simulink model "Galvo_sys_cc_neu_v32"  (R2013a)
settings: Solver=ode45  StartTime=0.0  StopTime=5e-3  MaxStep=1e-4  RelTol=1e-3  AbsTol=1e-5
PreLoadFcn:
  | paramCtrl=evalin('base','paramCtrl;');
  | 
  | I_LIM=str2num(paramCtrl.I_LIM);
  | Kbc=str2num(paramCtrl.Kbc);
InitFcn:
  | %I_LIM=str2num(paramCtrl.I_LIM);
  | %Kbc=str2num(paramCtrl.Kbc);
StartFcn:
  | %I_LIM=str2num(paramCtrl.I_LIM);
  | %Kbc=str2num(paramCtrl.Kbc);
values from neighbouring files (symbols this model uses):
  Lc = 170e-6    (= 0.00017)    [Galvo_process_analyze.m]
  Rc = 1.5    [Galvo_process_analyze.m]
undefined symbols (not defined in the file or in its folder): Rsh
libraries: simulink x2
settings Model: BufferReuse=off  Creator=mainster  LastModifiedBy=mainster
settings OptimizationCC: BlockReduction=off  OptimizeBlockIOStorage=off  BufferReuse=off  ExpressionFolding=off  LocalBlockOutputs=off
settings ModelReferenceCC: ModelReferenceNumInstancesAllowed=Single

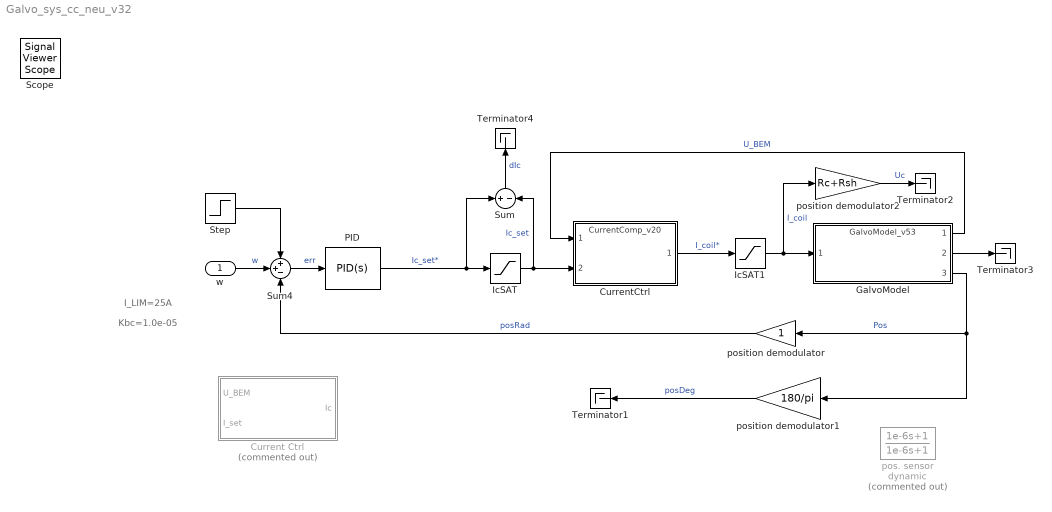
== system Galvo_sys_cc_neu_v32 ==
  note: I_LIM=25A
  note: Kbc=1.0e-05
  w : Inport
  Current Ctrl : Subsystem  Commented=on
  CurrentCtrl : ModelReference  ModelNameDialog=CurrentComp_v20.slx  SimulationMode=Normal  Variant=on  OverrideUsingVariant=cc_v20  ModelReferenceVersion=1.87  CopyOfModelName=CurrentComp_v20.slx  DefaultDataLogging=on
      mask Display:
      | str=sprintf('%s',get(gcbh,'ModelName'));
      | port_label('input', 2, 'I_{Set Coil}','texmode','on')
      | color('red');
      | port_label('input', 1, 'U_{BEM}','texmode','on')
      | color('black');
      | port_label('output', 1, 'I_{Coil}','texmode','on')
      | %text(.05,.98,['{\fontsize{12}\it\bf' strrep(str,'_',' ') '}'],'horizontalAlignment','left','verticalAlignment','top','texmode','on')
      | text(.95,0.95,['{\fontsize{12}\it\bfG_{cc}(s)}'],'horizontalAlignment','right','verticalAlignment','top','texmode','on')
      | %text(.15,.05,['{\fontsize{10}\itmechanics}'],'horizontalAlignment','left','verticalAlignment','bottom','texmode','on')
  GalvoModel : ModelReference  ModelNameDialog=GalvoModel_v53.slx  SimulationMode=Normal  Variant=on  OverrideUsingVariant=v53_neuer_cc  ModelReferenceVersion=1.60  CopyOfModelName=GalvoModel_v53.slx  DefaultDataLogging=on
      mask Display:
      | str=sprintf('%s',get(gcbh,'ModelName'));
      | port_label('input', 1, 'I_{Coil}','texmode','on')
      | color('blue');
      | port_label('output', 3, 'Pos','texmode','on')
      | color('black');
      | port_label('output', 2, 'Speed','texmode','on')
      | port_label('output', 1, 'U_{BEM}','texmode','on')
      | %text(.05,.98,['{\fontsize{12}\it\bf' strrep(str,'_',' ') '}'],'horizontalAlignment','left','verticalAlignment','top','texmode','on')
      | text(.015,.98,['{\fontsize{12}\it\bf' strrep(str,'_','\_') '}'],'horizontalAlignment','left','verticalAlignment','top','texmode','on')
      | text(.15,.05,['{\fontsize{10}\itmechanics}'],'horizontalAlignment','left','verticalAlignment','bottom','texmode','on')
  IcSAT : Saturate  UpperLimit=I_LIM  LowerLimit=-I_LIM
  IcSAT1 : Saturate  UpperLimit=I_LIM  LowerLimit=-I_LIM
  PID : simulink/Continuous/PID Controller  Controller=PID  TimeDomain=Continuous-time  SampleTime=1  IntegratorMethod=Forward Euler  FilterMethod=Forward Euler  Form=Ideal  P=0.582255500970855  I=10.299809554028  D=0.0214479671199487  N=4765.93232634932  InitialConditionSource=internal  InitialConditionForIntegrator=0  InitialConditionForFilter=0  ExternalReset=none  IgnoreLimit=on  LimitOutput=on  UpperSaturationLimit=I_LIM  LowerSaturationLimit=-I_LIM  LinearizeAsGain=off  AntiWindupMode=back-calculation  Kb=0.01  TrackingMode=off  Kt=0  PParamMin=[]  PParamMax=[]  IParamMin=[]  IParamMax=[]  DParamMin=[]  DParamMax=[]  NParamMin=[]  NParamMax=[]  KbParamMin=[]  KbParamMax=[]  KtParamMin=[]  KtParamMax=[]  POutMin=[]  POutMax=[]  IOutMin=[]  IOutMax=[]  DOutMin=[]  DOutMax=[]  NOutMin=[]  NOutMax=[]  KbOutMin=[]  KbOutMax=[]  KtOutMin=[]  KtOutMax=[]  IntegratorOutMin=[]  IntegratorOutMax=[]  FilterOutMin=[]  FilterOutMax=[]  SumOutMin=[]  SumOutMax=[]  SumI1OutMin=[]  SumI1OutMax=[]  SumI2OutMin=[]  SumI2OutMax=[]  SumI3OutMin=[]  SumI3OutMax=[]  SumDOutMin=[]  SumDOutMax=[]  SaturationOutMin=[]  SaturationOutMax=[]  IntegratorContinuousStateAttributes=''  IntegratorStateMustResolveToSignalObject=off  IntegratorRTWStateStorageClass=Auto  FilterContinuousStateAttributes=''  FilterStateMustResolveToSignalObject=off  FilterRTWStateStorageClass=Auto
      settings: AttributesFormatString=AWM=%<AntiWindupMode>\nD=%<D>\nI=%<I>\nN=%<N>\nP=%<P>\nLimit=+-%<UpperSaturationLimit>
  Step : Step  Time=1e-3  After=10*pi/180  SampleTime=0  ZeroCross=off
      settings: AttributesFormatString=Ampl.: %<After>
  Sum : Sum  Inputs=+-
  Sum4 : Sum  Inputs=++-
  Terminator{1..4} (4 alike) : Terminator
  pos. sensor dynamic : TransferFcn  Commented=on  Numerator=[1e-6 1]  Denominator=[1e-6 1]
  position demodulator : Gain
  position demodulator1 : Gain  Gain=180/pi
  position demodulator2 : Gain  Gain=Rc+Rsh
  Scope : SignalViewerScope  IOType=viewer  NumInputPorts=5  LegendLocations=|  RefreshTime=0.035000
      | 0.8137     0.89944     0.14296    0.057263
      | 0.85815     0.74553    0.098519    0.022346
      | 0.84926      0.5567     0.10741    0.022346
      | 0.82259     0.35154     0.13407    0.039804
      | 0.82259     0.16271     0.13407    0.039804
      settings: ShowLegends=on  TimeRange=0.005  YMin=-5~-10~-1~0~-5  YMax=20~30~1~0.2~15
  wires:
  Sum4/1 -> PID/1  "err"
  Step/1 -> Sum4/1
  w/1 -> Sum4/2  "w"
  position demodulator/1 -> Sum4/3  "posRad"
  GalvoModel/3 -> position demodulator/1, position demodulator1/1  "Pos"
  GalvoModel/1 -> CurrentCtrl/1  "U_BEM"
  PID/1 -> Sum/1, IcSAT/1  "Ic_set*"
  CurrentCtrl/1 -> IcSAT1/1  "I_coil*"
  position demodulator1/1 -> Terminator1/1  "posDeg"
  position demodulator2/1 -> Terminator2/1  "Uc"
  IcSAT/1 -> CurrentCtrl/2, Sum/2  "Ic_set"
  GalvoModel/2 -> Terminator3/1
  Sum/1 -> Terminator4/1  "dIc"
  IcSAT1/1 -> position demodulator2/1, GalvoModel/1  "I_coil"

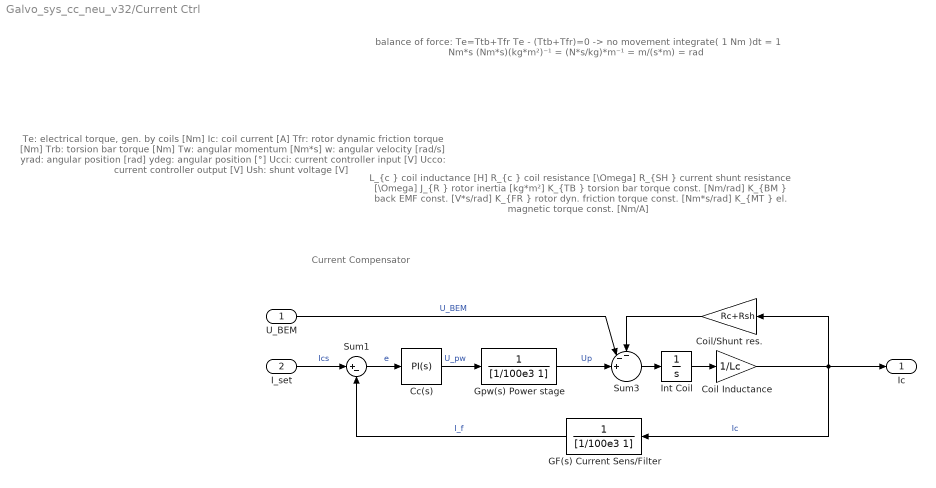
== system Galvo_sys_cc_neu_v32/Current Ctrl ==
  note: Current Compensator
  note: Te: 		electrical torque, gen. by coils		[Nm]
      |  Ic: 			coil current							[A]
      |  Tfr:		rotor dynamic friction torque 		[Nm]
      |  Trb:		torsion bar torque					[Nm]
      |  Tw:		angular momentum				[Nm*s]
      |  w:			angular velocity 					[rad/s]
      |  yrad:		angular position 					[rad]
      |  ydeg:		angular position 					[°]
      |  Ucci:		current controller input				[V]
      |  Ucco:		current controller output			[V]
      |  Ush:		shunt voltage						[V]
  note: L_{c  }	coil inductance 							[H]
      |  R_{c  }	coil resistance							[\Omega]
      |  R_{SH }	current shunt resistance				[\Omega]
      |  J_{R  }	rotor inertia 							[kg*m²]
      |  K_{TB }	torsion bar torque const. 			[Nm/rad]
      |  K_{BM }	back EMF const.							[V*s/rad]
      |  K_{FR }	rotor dyn. friction torque const.	[Nm*s/rad]
      |  K_{MT }	el. magnetic torque const.			[Nm/A]
  note: balance of force: 	Te=Ttb+Tfr
      | 					Te - (Ttb+Tfr)=0  ->  no movement
      |
      |  integrate( 1 Nm )dt = 1 Nm*s
      |  (Nm*s)(kg*m²)⁻¹ = (N*s/kg)*m⁻¹ = m/(s*m) = rad
  U_BEM : Inport
  I_set : Inport  Port=2
  Cc(s) : simulink/Continuous/PID Controller  Controller=PI  TimeDomain=Continuous-time  SampleTime=1  IntegratorMethod=Forward Euler  FilterMethod=Forward Euler  Form=Ideal  P=2.58986900309333  I=14540.01765706  D=0  N=100  InitialConditionSource=internal  InitialConditionForIntegrator=0  InitialConditionForFilter=0  ExternalReset=none  LimitOutput=off  UpperSaturationLimit=inf  LowerSaturationLimit=-inf  LinearizeAsGain=on  AntiWindupMode=none  Kb=1  TrackingMode=off  Kt=1  PParamMin=[]  PParamMax=[]  IParamMin=[]  IParamMax=[]  DParamMin=[]  DParamMax=[]  NParamMin=[]  NParamMax=[]  KbParamMin=[]  KbParamMax=[]  KtParamMin=[]  KtParamMax=[]  POutMin=[]  POutMax=[]  IOutMin=[]  IOutMax=[]  DOutMin=[]  DOutMax=[]  NOutMin=[]  NOutMax=[]  KbOutMin=[]  KbOutMax=[]  KtOutMin=[]  KtOutMax=[]  IntegratorOutMin=[]  IntegratorOutMax=[]  FilterOutMin=[]  FilterOutMax=[]  SumOutMin=[]  SumOutMax=[]  SumI1OutMin=[]  SumI1OutMax=[]  SumI2OutMin=[]  SumI2OutMax=[]  SumI3OutMin=[]  SumI3OutMax=[]  SumDOutMin=[]  SumDOutMax=[]  SaturationOutMin=[]  SaturationOutMax=[]  IntegratorContinuousStateAttributes=''  IntegratorStateMustResolveToSignalObject=off  IntegratorRTWStateStorageClass=Auto  FilterContinuousStateAttributes=''  FilterStateMustResolveToSignalObject=off  FilterRTWStateStorageClass=Auto
  Coil Inductance : Gain  Gain=1/Lc
  Coil/Shunt res. : Gain  Gain=Rc+Rsh
  GF(s) Current Sens/Filter : TransferFcn  Denominator=[1/100e3 1]
  Gpw(s) Power stage : TransferFcn  Denominator=[1/100e3 1]
  Int Coil : Integrator
  Sum1 : Sum  Inputs=|+-
  Sum3 : Sum  Inputs=--+||
  Ic : Outport
  wires:
  Cc(s)/1 -> Gpw(s) Power stage/1  "U_pw"
  GF(s) Current Sens/Filter/1 -> Sum1/2  "I_f"
  Coil/Shunt res./1 -> Sum3/1
  Sum3/1 -> Int Coil/1
  Gpw(s) Power stage/1 -> Sum3/3  "Up"
  Coil Inductance/1 -> Ic/1, GF(s) Current Sens/Filter/1, Coil/Shunt res./1  "Ic"
  I_set/1 -> Sum1/1  "Ics"
  Sum1/1 -> Cc(s)/1  "e"
  Int Coil/1 -> Coil Inductance/1
  U_BEM/1 -> Sum3/2  "U_BEM"
